simulink model "lab6"  (R2022b)
settings: Solver=VariableStepAuto  StartTime=0.0  StopTime=40  RelTol=1e-3
undefined symbols (not defined in the file): a, b, c, d, k, P, T, Td, Ti
settings Model: Creator=dambi  LastModifiedBy=dambi

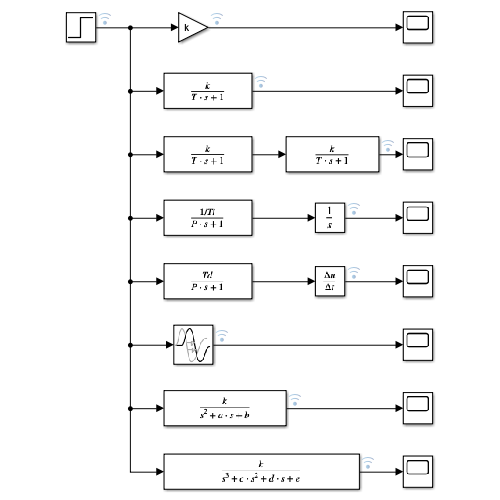
[thumbnail: Simulink's stored preview of the top-level diagram]
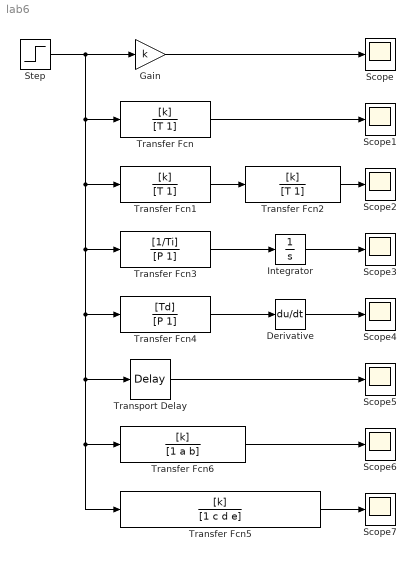
== system lab6 ==
  Derivative : Derivative
  Gain : Gain  Gain=k
  Integrator : Integrator
  Scope{,1..7} (8 alike) : Scope
  Step : Step  SampleTime=0
  Transfer Fcn : TransferFcn  Numerator=[k]  Denominator=[T 1]
  Transfer Fcn1 : TransferFcn  Numerator=[k]  Denominator=[T 1]
  Transfer Fcn2 : TransferFcn  Numerator=[k]  Denominator=[T 1]
  Transfer Fcn3 : TransferFcn  Numerator=[1/Ti]  Denominator=[P 1]
  Transfer Fcn4 : TransferFcn  Numerator=[Td]  Denominator=[P 1]
  Transfer Fcn5 : TransferFcn  Numerator=[k]  Denominator=[1 c d e]
  Transfer Fcn6 : TransferFcn  Numerator=[k]  Denominator=[1 a b]
  Transport Delay : TransportDelay
  wires:
  Transfer Fcn1/1 -> Transfer Fcn2/1
  Transfer Fcn4/1 -> Derivative/1
  Transfer Fcn3/1 -> Integrator/1
  Gain/1 -> Scope/1
  Transfer Fcn/1 -> Scope1/1
  Transfer Fcn2/1 -> Scope2/1
  Integrator/1 -> Scope3/1
  Derivative/1 -> Scope4/1
  Transport Delay/1 -> Scope5/1
  Transfer Fcn6/1 -> Scope6/1
  Transfer Fcn5/1 -> Scope7/1
  Step/1 -> Gain/1, Transfer Fcn/1, Transfer Fcn1/1, Transfer Fcn3/1, Transfer Fcn4/1, Transport Delay/1, Transfer Fcn6/1, Transfer Fcn5/1
